simulink model "RoBee_model"  (R2021b)
settings: Solver=VariableStepAuto  StartTime=0.0  StopTime=10.0  RelTol=1e-3
undefined symbols (not defined in the file): additional_weight, weight_torso, X, Y, Z
libraries: sm_lib x31, nesl_utility x11
(part 2 of 2)

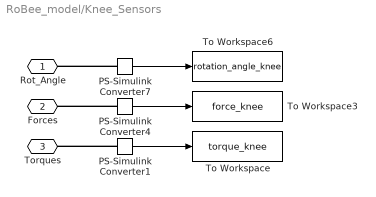
== system RoBee_model/Knee_Sensors ==
  PS-Simulink Converter1 : nesl_utility/PS-Simulink Converter  PhysicalDomain=network_engine_domain  SubClassName=ps_output  LeftPortType=input  RightPortType=output  PseudoPeriodic=off  Frequencies=[]  Unit=inherit  AffineConversion=off
      settings: SourceProductBaseCode=PW,SS
  PS-Simulink Converter4 : nesl_utility/PS-Simulink Converter  PhysicalDomain=network_engine_domain  SubClassName=ps_output  LeftPortType=input  RightPortType=output  PseudoPeriodic=off  Frequencies=[]  Unit=inherit  AffineConversion=off
      settings: SourceProductBaseCode=PW,SS
  PS-Simulink Converter7 : nesl_utility/PS-Simulink Converter  PhysicalDomain=network_engine_domain  SubClassName=ps_output  LeftPortType=input  RightPortType=output  PseudoPeriodic=off  Frequencies=[]  Unit=inherit  AffineConversion=off
      settings: SourceProductBaseCode=PW,SS
  To Workspace : ToWorkspace  VariableName=torque_knee  SaveFormat=Timeseries  SampleTime=-1
  To Workspace3 : ToWorkspace  VariableName=force_knee  SaveFormat=Timeseries  SampleTime=-1
  To Workspace6 : ToWorkspace  VariableName=rotation_angle_knee  SaveFormat=Timeseries  SampleTime=-1
  Rot_Angle : PMIOPort  Side=Left
  Forces : PMIOPort  Port=2  Side=Left
  Torques : PMIOPort  Port=3  Side=Left
  wires:
  PS-Simulink Converter4/1 -> To Workspace3/1
  PS-Simulink Converter7/1 -> To Workspace6/1
  PS-Simulink Converter1/1 -> To Workspace/1
  connections:
  PS-Simulink Converter1/LConn1 -- Torques/RConn1
  PS-Simulink Converter4/LConn1 -- Forces/RConn1
  PS-Simulink Converter7/LConn1 -- Rot_Angle/RConn1
